simulink model "winkelberechnung"  (R2023a)
settings: Solver=VariableStepAuto  StartTime=0.0  StopTime=10.0  RelTol=1e-3
settings Model: Creator=hp  LastModifiedBy=hp

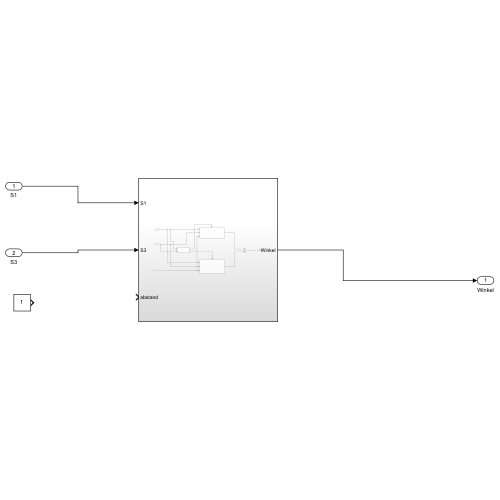
[thumbnail: Simulink's stored preview of the top-level diagram]
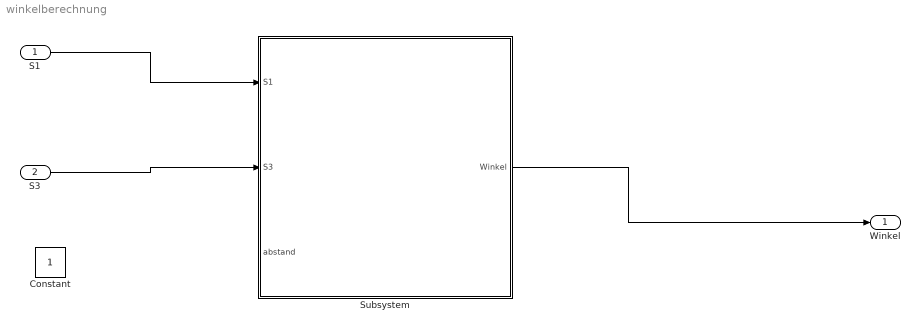
== system winkelberechnung ==
  S1 : Inport
  S3 : Inport  Port=2
  Constant : Constant
  Subsystem : Subsystem
  Winkel : Outport
  wires:
  S1/1 -> Subsystem/1(S1)
  S3/1 -> Subsystem/2(S3)
  Subsystem/1(Winkel) -> Winkel/1

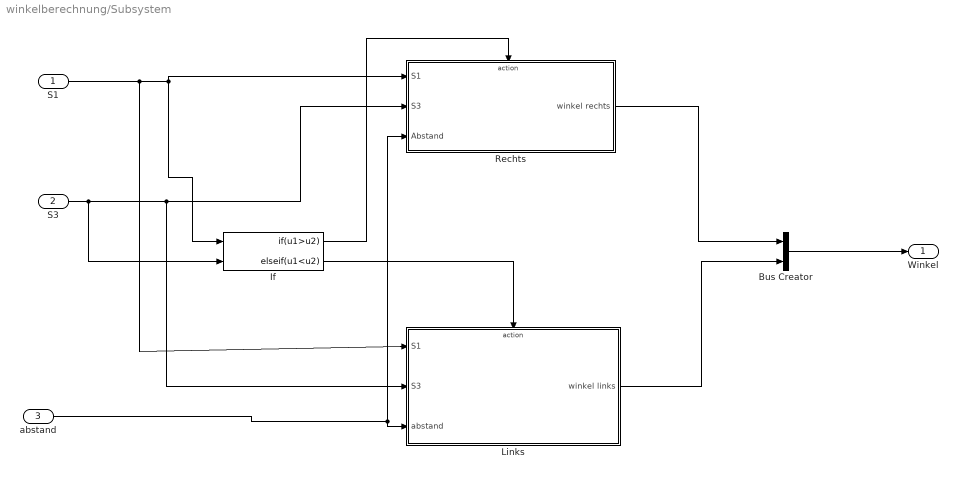
== system winkelberechnung/Subsystem ==
  S1 : Inport
  S3 : Inport  Port=2
  abstand : Inport  Port=3
  Bus Creator : BusCreator  Inputs=2
  If : If  NumInputs=2  IfExpression=u1>u2  ElseIfExpressions=u1<u2  ShowElse=off
  Links : Subsystem  TreatAsAtomicUnit=on
  Rechts : Subsystem  TreatAsAtomicUnit=on
  Winkel : Outport
  wires:
  S1/1 -> Links/1(S1), If/1, Rechts/1(S1)
  Rechts/1(winkel rechts) -> Bus Creator/1
  If/1 -> Rechts/Action
  S3/1 -> If/2, Links/2(S3), Rechts/2(S3)
  abstand/1 -> Rechts/3(Abstand), Links/3(abstand)
  Bus Creator/1 -> Winkel/1
  If/2 -> Links/Action
  Links/1(winkel links) -> Bus Creator/2

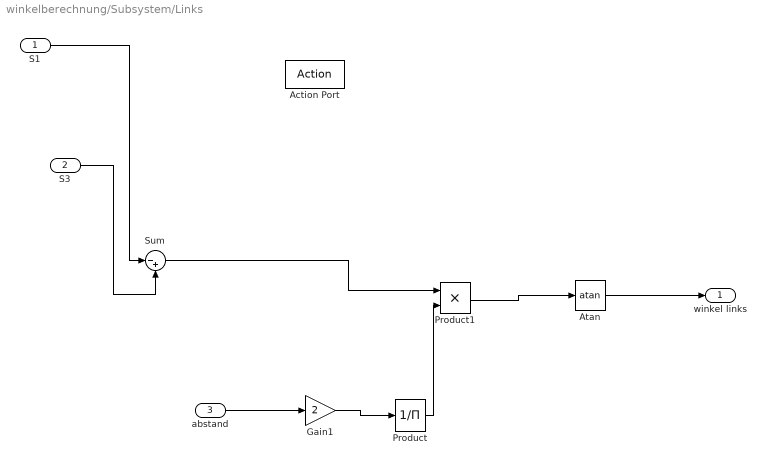
== system winkelberechnung/Subsystem/Links ==
  S1 : Inport
  S3 : Inport  Port=2
  abstand : Inport  Port=3
  Action Port : ActionPort  ActionPortLabel=elseif(u1<u2)
  Atan : Trigonometry  Operator=atan
  Gain1 : Gain  Gain=2
  Product : Product  Inputs=/
  Product1 : Product
  Sum : Sum  Inputs=|-+
  winkel links : Outport
  wires:
  S1/1 -> Sum/1
  Product/1 -> Product1/2
  S3/1 -> Sum/2
  Atan/1 -> winkel links/1
  Product1/1 -> Atan/1
  Sum/1 -> Product1/1
  Gain1/1 -> Product/1
  abstand/1 -> Gain1/1

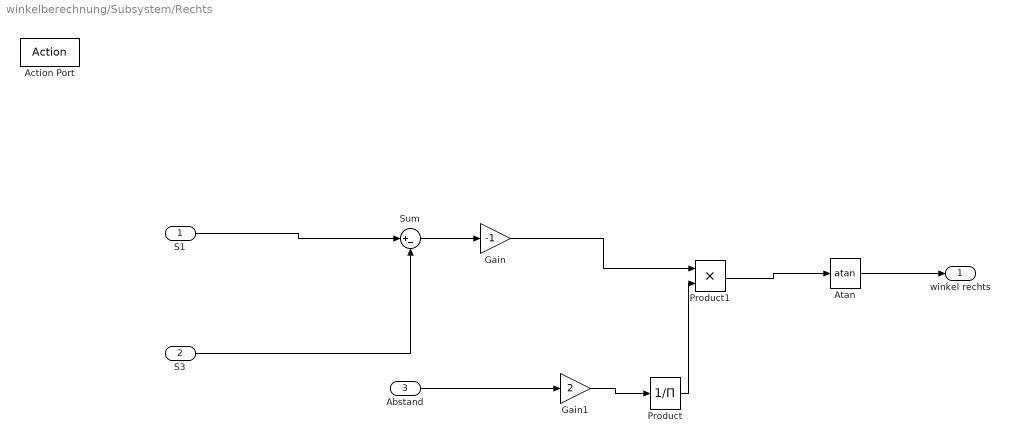
== system winkelberechnung/Subsystem/Rechts ==
  S1 : Inport
  S3 : Inport  Port=2
  Abstand : Inport  Port=3
  Action Port : ActionPort  ActionPortLabel=if(u1>u2)
  Atan : Trigonometry  Operator=atan
  Gain : Gain  Gain=-1
  Gain1 : Gain  Gain=2
  Product : Product  Inputs=/
  Product1 : Product
  Sum : Sum  Inputs=|+-
  winkel rechts : Outport
  wires:
  S3/1 -> Sum/2
  Sum/1 -> Gain/1
  Atan/1 -> winkel rechts/1
  S1/1 -> Sum/1
  Product1/1 -> Atan/1
  Gain1/1 -> Product/1
  Gain/1 -> Product1/1
  Product/1 -> Product1/2
  Abstand/1 -> Gain1/1
